simulink model "test_conv2d"  (R2017a)
settings: Solver=FixedStepDiscrete  StartTime=0.0  StopTime=1  FixedStep=1  RelTol=1e-3
undefined symbols (not defined in the file or in its folder): gray
libraries: ad_blocks x1, visionsources x1, visiongeotforms x1
settings Model: Creator=eruffaldi  LastModifiedBy=eruffaldi

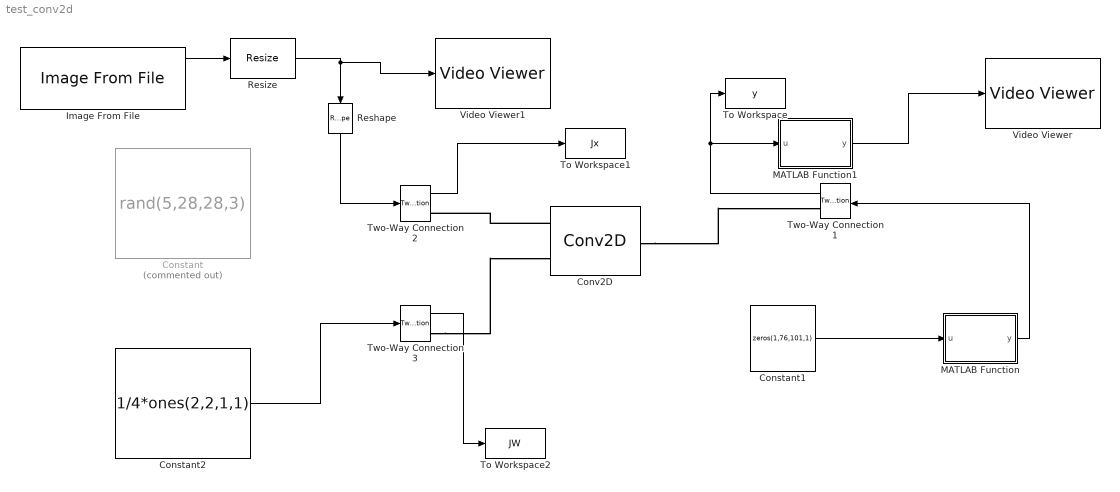
== system test_conv2d ==
  Constant : Constant  Commented=on  Value=rand(5,28,28,3)
  Constant1 : Constant  Value=zeros(1,76,101,1)
  Constant2 : Constant  Value=1/4*ones(2,2,1,1)
  Conv2D : ad_blocks/Conv2D  stride=[1,2,2,1]
  Image From File : visionsources/Image From File  Tag=vipblks_nd  FileName=peppers.png  imagePorts=Separate color signals  Ts=inf  ImageDataType=double  Signed=on  WordLength=16  sdImageDataType=uint(8)  FractionLengthMode=User-defined  FractionLength=15  OutPortLabels=R|G|B
      settings: SourceProductName=Computer Vision System Toolbox
  MATLAB Function : MATLAB Function  TreatAsAtomicUnit=on
  MATLAB Function1 : MATLAB Function  TreatAsAtomicUnit=on
  Reshape : Reshape  OutputDimensionality=Customize  OutputDimensions=[1,75,100,1]
  Resize : visiongeotforms/Resize  specify=Number of output columns and preserve aspect ratio  rfactor=[200 150]  outCols=100  outRows=25  outRowsCols=[25 35]  interp_method=Bilinear  antialias=on  useROI=off  roiFlag=off  prodOutputMode=Binary point scaling  prodOutputWordLength=32  prodOutputFracLength=10  roundingMode=Nearest  overflowMode=on
      settings: SourceProductName=Computer Vision System Toolbox  SourceProductBaseCode=VP
  To Workspace : ToWorkspace  VariableName=y  SaveFormat=Timeseries  SampleTime=-1
  To Workspace1 : ToWorkspace  VariableName=Jx  SaveFormat=Timeseries  SampleTime=-1
  To Workspace2 : ToWorkspace  VariableName=JW  SaveFormat=Timeseries  SampleTime=-1
  Two-Way Connection1 : TwoWayConnection
  Two-Way Connection2 : TwoWayConnection
  Two-Way Connection3 : TwoWayConnection
  Video Viewer : VideoViewer  colormapValue=gray(256)  FigPos=[1 894 1440 774]
  Video Viewer1 : VideoViewer  colormapValue=gray(256)  FigPos=[511 601 418 304]
  wires:
  MATLAB Function/1(y) -> Two-Way Connection1/1
  Two-Way Connection1/1 -> MATLAB Function1/1(u), To Workspace/1
  Two-Way Connection2/1 -> To Workspace1/1
  Constant1/1 -> MATLAB Function/1(u)
  Two-Way Connection3/1 -> To Workspace2/1
  Constant2/1 -> Two-Way Connection3/1
  Image From File/1 -> Resize/1
  Resize/1 -> Video Viewer1/1, Reshape/1
  Reshape/1 -> Two-Way Connection2/1
  MATLAB Function1/1(y) -> Video Viewer/1
  connections:
  Conv2D/RConn1 -- Two-Way Connection1/RConn1
  Conv2D/LConn1 -- Two-Way Connection2/RConn1
  Two-Way Connection3/RConn1 -- Conv2D/LConn2

== matlab function test_conv2d/MATLAB Function1 ==
  data: y output; u input
function y = fcn(u)
y = squeeze(u(1,:,:,1));

== matlab function test_conv2d/MATLAB Function ==
  data: y output; u input
function y = fcn(u)
y = u;
y(:) = 1:numel(y);
